simulink model "nlmodel_3D"  (R2022b)
settings: Solver=ode45  StartTime=0.0  StopTime=50  RelTol=1e-3  EnableMultiTasking=on
values from neighbouring files (symbols this model uses):
  eps0 = 0    [nl_parameters_3D.m]
  eps0dot = 0    [nl_parameters_3D.m]
  lam0 = 0    [nl_parameters_3D.m]
  lam0dot = 0    [nl_parameters_3D.m]
  p1 = (-(Mf+Mb)*g*La+Mc*g*Lc)/Jeps    (= -1.5604744186)    [nl_parameters_3D.m]
  p10 = -Km*La/Jlam    (= -0.0907317073171)    [nl_parameters_3D.m]
  p2 = (-(Mf+Mb)*g*(Ld+Le)+Mc*g*Ld)/Jeps    (= -0.169963953488)    [nl_parameters_3D.m]
  p3 = -Neps/Jeps    (= -0.00116279069767)    [nl_parameters_3D.m]
  p4 = Km*La/Jeps    (= 0.086511627907)    [nl_parameters_3D.m]
  p5 = (-Mf+Mb)*g*Lh/Jro    (= 0)    [nl_parameters_3D.m]
  p6 = -(Mf+Mb)*g*Le/Jro    (= -6.33190909091)    [nl_parameters_3D.m]
  p7 = -Nro/Jro    (= -0.0227272727273)    [nl_parameters_3D.m]
  p8 = Km*Lh/Jro    (= 0.490909090909)    [nl_parameters_3D.m]
  p9 = -Nlam/Jlam    (= -0.00609756097561)    [nl_parameters_3D.m]
  ro0 = 0    [nl_parameters_3D.m]
  ro0dot = 0    [nl_parameters_3D.m]
  Vb0 = u0(2)    [nl_parameters_3D.m]
  Vf0 = u0(1)    [nl_parameters_3D.m]
settings Model: Creator=giusgiordano  LastModifiedBy=abdul
settings SolverCC: AlgebraicLoopSolver=TrustRegion
settings DataIOCC: LimitDataPoints=on  SaveFormat=Array  SignalLoggingSaveFormat=ModelDataLogs  ReturnWorkspaceOutputs=off
settings OptimizationCC: ExpressionDepthLimit=2147483647  LifeSpan=inf
settings DebuggingCC: UnderspecifiedInitializationDetection=Classic  MergeDetectMultiDrivingBlocksExec=none  SolverPrmCheckMsg=warning  FcnCallInpInsideContextMsg=warning  UnconnectedInputMsg=warning  UnconnectedOutputMsg=warning  UnconnectedLineMsg=warning  StateNameClashWarn=warning  SFUnexpectedBacktrackingDiag=warning  SFNoUnconditionalDefaultTransitionDiag=warning  SFExecutionAtInitializationDiag=none  SFMachineParentedDataDiag=warning  ArithmeticOperatorsInVariantConditions=warning
settings HardwareCC: ProdBitPerPointer=32  ProdBitPerSizeT=32  ProdBitPerPtrDiffT=32  ProdLargestAtomicFloat=None  ProdIntDivRoundTo=Undefined  ProdEndianess=Unspecified  ProdWordSize=32  ProdHWDeviceType=32-bit Generic
settings ModelReferenceCC: PropagateSignalLabelsOutOfModel=off
settings SFSimCC: SimUseLocalCustomCode=off  CustomCodeUndefinedFunction=UseInterfaceOnly
settings RTWCC: RTWUseLocalCustomCode=off
settings CodeAppCC: StateflowObjectComments=on
settings GRTTargetCC: TargetLangStandard=C89/C90 (ANSI)  CombineOutputUpdateFcns=off  GRTInterface=on
settings ConfigComp: CovMetricSettings=dw  CovSaveCumulativeToWorkspaceVar=on  CovSaveSingleToWorkspaceVar=on  CovExternalEMLEnable=off

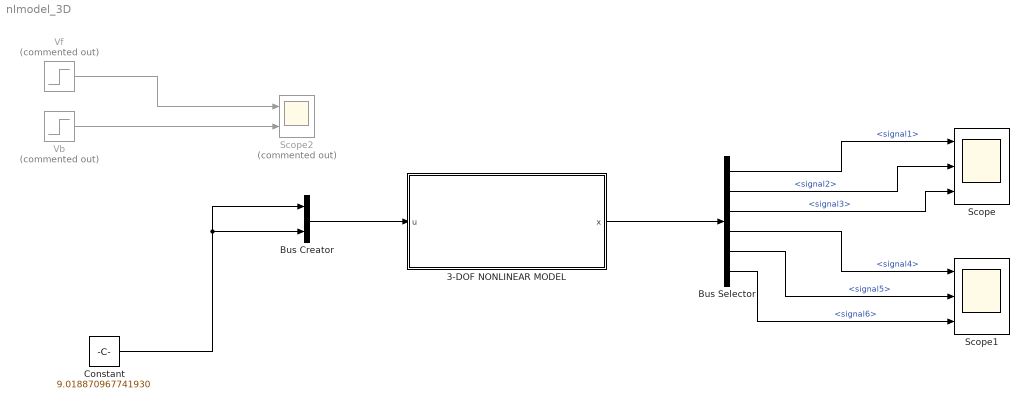
== system nlmodel_3D ==
  3-DOF NONLINEAR MODEL : Subsystem
  Bus Creator : BusCreator  Inputs=2
  Bus Selector : BusSelector  OutputSignals=signal1,signal2,signal3,signal4,signal5,signal6
  Constant : Constant  Value=9.018870967741930
  Scope : Scope  NumInputPorts=3
  Scope1 : Scope  NumInputPorts=3
  Scope2 : Scope  Commented=on  NumInputPorts=2
  Vb : Step  Commented=on  Time=0  After=Vb0  SampleTime=0
  Vf : Step  Commented=on  Time=0  After=Vf0  SampleTime=0
  wires:
  3-DOF NONLINEAR MODEL/1(x) -> Bus Selector/1
  Bus Creator/1 -> 3-DOF NONLINEAR MODEL/1(u)
  Vf/1 -> Scope2/1
  Vb/1 -> Scope2/2
  Bus Selector/1 -> Scope/1  "<signal1>"
  Bus Selector/2 -> Scope/2  "<signal2>"
  Bus Selector/3 -> Scope/3  "<signal3>"
  Bus Selector/4 -> Scope1/1  "<signal4>"
  Bus Selector/5 -> Scope1/2  "<signal5>"
  Bus Selector/6 -> Scope1/3  "<signal6>"
  Constant/1 -> Bus Creator/2, Bus Creator/1

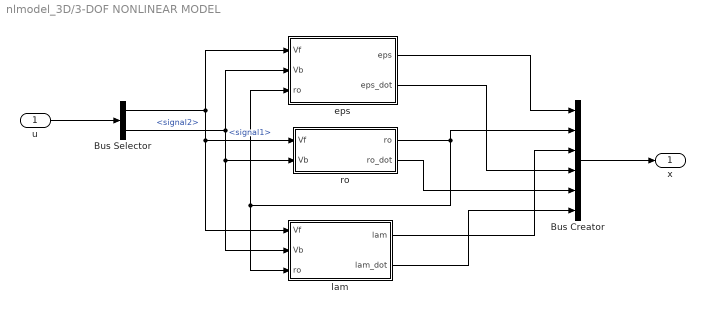
== system nlmodel_3D/3-DOF NONLINEAR MODEL ==
  u : Inport
  Bus Creator : BusCreator  Inputs=6
  Bus Selector : BusSelector  OutputSignals=signal1,signal2
  eps : Subsystem
  lam : Subsystem
  ro : Subsystem
  x : Outport
  wires:
  u/1 -> Bus Selector/1
  Bus Selector/1 -> eps/1(Vf), ro/1(Vf), lam/1(Vf)  "<signal1>"
  Bus Selector/2 -> eps/2(Vb), ro/2(Vb), lam/2(Vb)  "<signal2>"
  ro/1(ro) -> Bus Creator/2, eps/3(ro), lam/3(ro)
  Bus Creator/1 -> x/1
  eps/1(eps) -> Bus Creator/1
  lam/1(lam) -> Bus Creator/3
  eps/2(eps_dot) -> Bus Creator/4
  ro/2(ro_dot) -> Bus Creator/5
  lam/2(lam_dot) -> Bus Creator/6

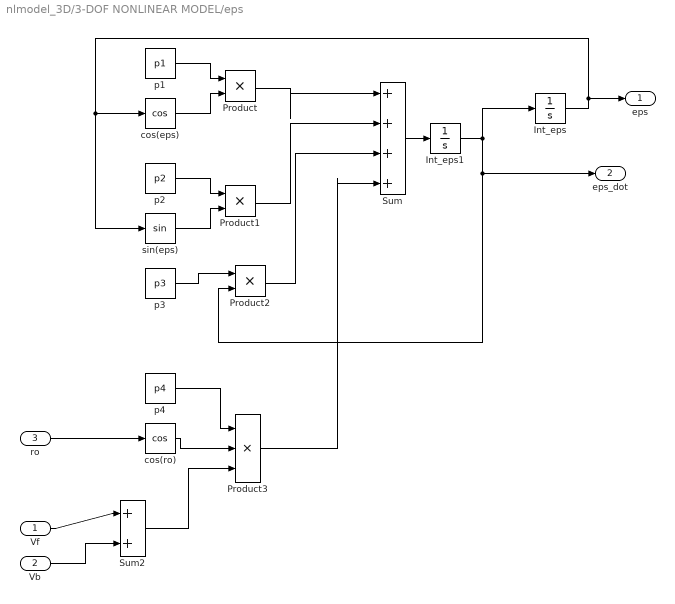
== system nlmodel_3D/3-DOF NONLINEAR MODEL/eps ==
  Vf : Inport
  Vb : Inport  Port=2
  ro : Inport  Port=3
  Int_eps : Integrator  InitialCondition=eps0  ContinuousStateAttributes='eps'
  Int_eps1 : Integrator  InitialCondition=eps0dot  ContinuousStateAttributes='epsdot'
  Product : Product  RndMeth=Zero
  Product1 : Product  RndMeth=Zero
  Product2 : Product  RndMeth=Zero
  Product3 : Product  Inputs=3  RndMeth=Zero
  Sum : Sum  Inputs=|++++
  Sum2 : Sum  Inputs=|++
  cos(eps) : Trigonometry  Operator=cos
  cos(ro) : Trigonometry  Operator=cos
  p1 : Constant  Value=p1
  p2 : Constant  Value=p2
  p3 : Constant  Value=p3
  p4 : Constant  Value=p4
  sin(eps) : Trigonometry
  eps : Outport
  eps_dot : Outport  Port=2
  wires:
  Int_eps/1 -> cos(eps)/1, sin(eps)/1, eps/1
  p1/1 -> Product/1
  cos(eps)/1 -> Product/2
  Product/1 -> Sum/1
  p2/1 -> Product1/1
  sin(eps)/1 -> Product1/2
  Product1/1 -> Sum/2
  p3/1 -> Product2/1
  Product2/1 -> Sum/3
  p4/1 -> Product3/1
  cos(ro)/1 -> Product3/2
  ro/1 -> cos(ro)/1
  Product3/1 -> Sum/4
  Sum/1 -> Int_eps1/1
  Int_eps1/1 -> Product2/2, eps_dot/1, Int_eps/1
  Vf/1 -> Sum2/1
  Vb/1 -> Sum2/2
  Sum2/1 -> Product3/3

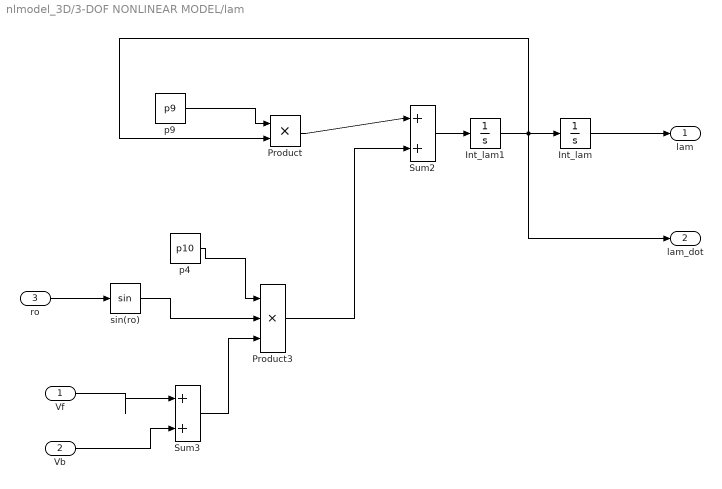
== system nlmodel_3D/3-DOF NONLINEAR MODEL/lam ==
  Vf : Inport
  Vb : Inport  Port=2
  ro : Inport  Port=3
  Int_lam : Integrator  InitialCondition=lam0  ContinuousStateAttributes='lam'
  Int_lam1 : Integrator  InitialCondition=lam0dot  ContinuousStateAttributes='lamdot'
  Product : Product  RndMeth=Zero
  Product3 : Product  Inputs=3  RndMeth=Zero
  Sum2 : Sum  Inputs=|++
  Sum3 : Sum  Inputs=|++
  p4 : Constant  Value=p10
  p9 : Constant  Value=p9
  sin(ro) : Trigonometry
  lam : Outport
  lam_dot : Outport  Port=2
  wires:
  Int_lam/1 -> lam/1
  p9/1 -> Product/1
  p4/1 -> Product3/1
  sin(ro)/1 -> Product3/2
  ro/1 -> sin(ro)/1
  Product/1 -> Sum2/1
  Sum2/1 -> Int_lam1/1
  Product3/1 -> Sum2/2
  Int_lam1/1 -> lam_dot/1, Product/2, Int_lam/1
  Vf/1 -> Sum3/1
  Vb/1 -> Sum3/2
  Sum3/1 -> Product3/3

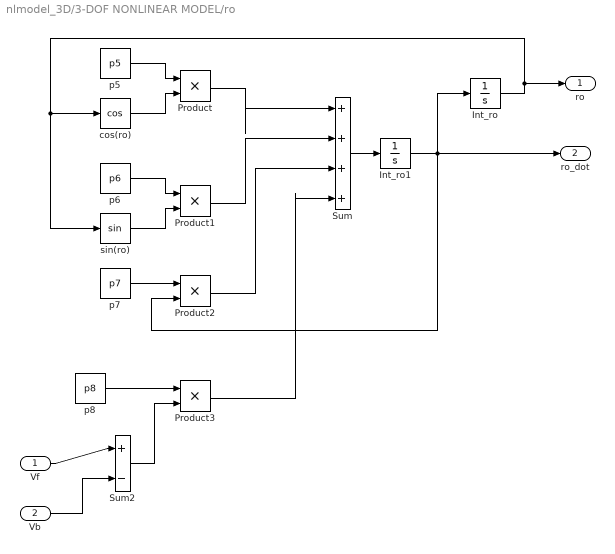
== system nlmodel_3D/3-DOF NONLINEAR MODEL/ro ==
  Vf : Inport
  Vb : Inport  Port=2
  Int_ro : Integrator  InitialCondition=ro0  ContinuousStateAttributes='ro'
  Int_ro1 : Integrator  InitialCondition=ro0dot  ContinuousStateAttributes='rodot'
  Product{,1..3} (4 alike) : Product  RndMeth=Zero
  Sum : Sum  Inputs=|++++
  Sum2 : Sum  Inputs=|+-
  cos(ro) : Trigonometry  Operator=cos
  p5 : Constant  Value=p5
  p6 : Constant  Value=p6
  p7 : Constant  Value=p7
  p8 : Constant  Value=p8
  sin(ro) : Trigonometry
  ro : Outport
  ro_dot : Outport  Port=2
  wires:
  Int_ro/1 -> cos(ro)/1, sin(ro)/1, ro/1
  p5/1 -> Product/1
  cos(ro)/1 -> Product/2
  Product/1 -> Sum/1
  p6/1 -> Product1/1
  sin(ro)/1 -> Product1/2
  Product1/1 -> Sum/2
  p7/1 -> Product2/1
  Product2/1 -> Sum/3
  p8/1 -> Product3/1
  Product3/1 -> Sum/4
  Int_ro1/1 -> Product2/2, ro_dot/1, Int_ro/1
  Sum/1 -> Int_ro1/1
  Vf/1 -> Sum2/1
  Vb/1 -> Sum2/2
  Sum2/1 -> Product3/2
